simulink model "evaporator_no_subs"  (R2018b)
settings: Solver=VariableStepAuto  StartTime=0.0  StopTime=10.0  RelTol=1e-3
settings Model: Creator=jh2044  LastModifiedBy=jh2044

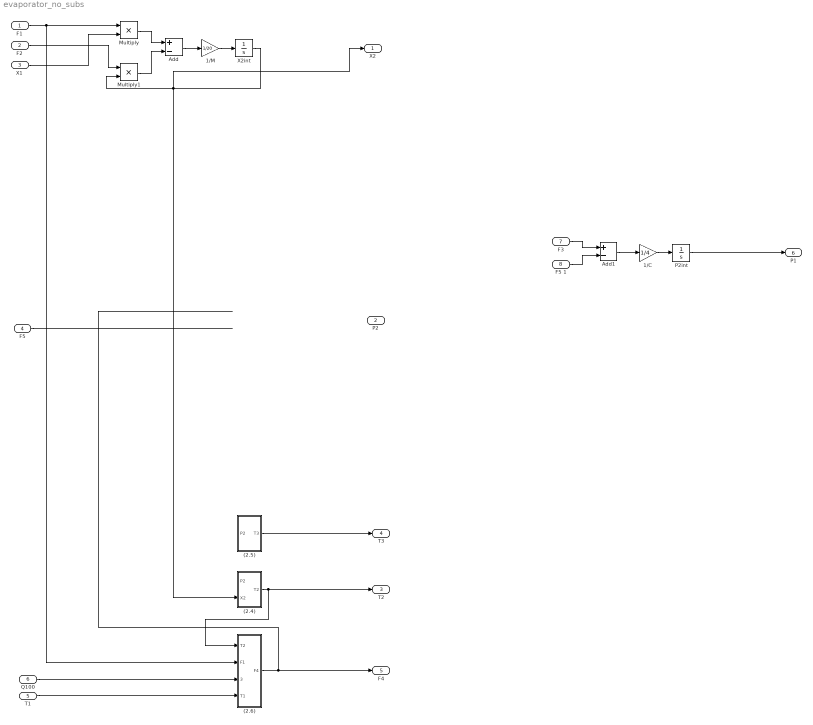
== system evaporator_no_subs ==
  F1 : Inport
  F2 : Inport  Port=2
  X1 : Inport  Port=3
  "F5 " : Inport  Port=4
  T1 : Inport  Port=5
  Q100 : Inport  Port=6
  F3 : Inport  Port=7
  F5 1 : Inport  Port=8
  (2.4) : Subsystem
  (2.5) : Subsystem
  (2.6) : Subsystem
  1/C : Gain  Gain=1/4
  1/M : Gain  Gain=1/20
  Add : Sum  Inputs=+-
  Add1 : Sum  Inputs=+-
  Multiply : Product
  Multiply1 : Product
  P2int : Integrator
  X2int : Integrator
  "X2 " : Outport
  P2 : Outport  Port=2
  T2 : Outport  Port=3
  T3 : Outport  Port=4
  F4 : Outport  Port=5
  P1 : Outport  Port=6
  wires:
  (2.4)/1(T2) -> (2.6)/1(T2), T2/1
  "F5 "/1 -> ?
  T1/1 -> (2.6)/4(T1)
  (2.6)/1(F4) -> F4/1
  (2.5)/1(T3) -> T3/1
  Q100/1 -> (2.6)/3(Q100)
  F1/1 -> (2.6)/2(F1), Multiply/1
  ? -> P2/1, (2.4)/1(P2), (2.5)/1(P2)
  1/M/1 -> X2int/1
  Multiply/1 -> Add/1
  X2int/1 -> (2.4)/2(X2), Multiply1/2, "X2 "/1
  F2/1 -> Multiply1/1
  X1/1 -> Multiply/2
  Add/1 -> 1/M/1
  Multiply1/1 -> Add/2
  Add1/1 -> 1/C/1
  1/C/1 -> P2int/1
  F5 1/1 -> Add1/2
  F3/1 -> Add1/1
  P2int/1 -> P1/1

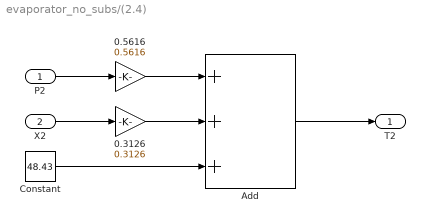
== system evaporator_no_subs/(2.4) ==
  P2 : Inport
  X2 : Inport  Port=2
  0.3126 : Gain  Gain=0.3126
  0.5616 : Gain  Gain=0.5616
  Add : Sum  Inputs=+++
  Constant : Constant  Value=48.43
  T2 : Outport
  wires:
  Constant/1 -> Add/3
  X2/1 -> 0.3126/1
  P2/1 -> 0.5616/1
  0.3126/1 -> Add/2
  0.5616/1 -> Add/1
  Add/1 -> T2/1

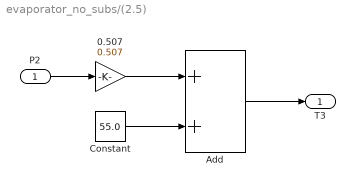
== system evaporator_no_subs/(2.5) ==
  P2 : Inport
  0.507 : Gain  Gain=0.507
  Add : Sum
  Constant : Constant  Value=55.0
  T3 : Outport
  wires:
  0.507/1 -> Add/1
  Add/1 -> T3/1
  Constant/1 -> Add/2
  P2/1 -> 0.507/1

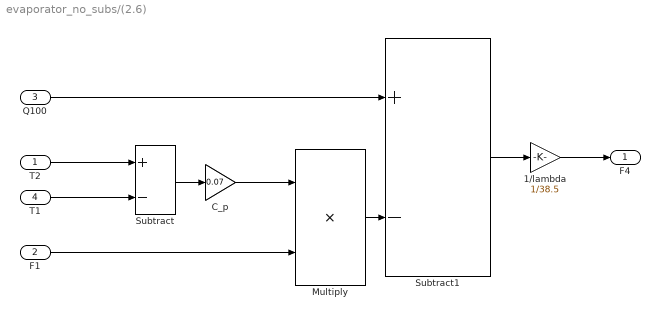
== system evaporator_no_subs/(2.6) ==
  T2 : Inport
  F1 : Inport  Port=2
  Q100 : Inport  Port=3
  T1 : Inport  Port=4
  1/lambda : Gain  Gain=1/38.5
  C_p : Gain  Gain=0.07
  Multiply : Product
  Subtract : Sum  Inputs=+-
  Subtract1 : Sum  Inputs=+-
  F4 : Outport
  wires:
  1/lambda/1 -> F4/1
  T2/1 -> Subtract/1
  Q100/1 -> Subtract1/1
  F1/1 -> Multiply/2
  Multiply/1 -> Subtract1/2
  Subtract1/1 -> 1/lambda/1
  C_p/1 -> Multiply/1
  T1/1 -> Subtract/2
  Subtract/1 -> C_p/1
